simulink model "PedalBoard"  (R2018b)
settings: Solver=VariableStepAuto  StartTime=0.0  StopTime=10.0  RelTol=1e-3
libraries: canoelib x4
settings Model: Creator=jackb  LastModifiedBy=jackb

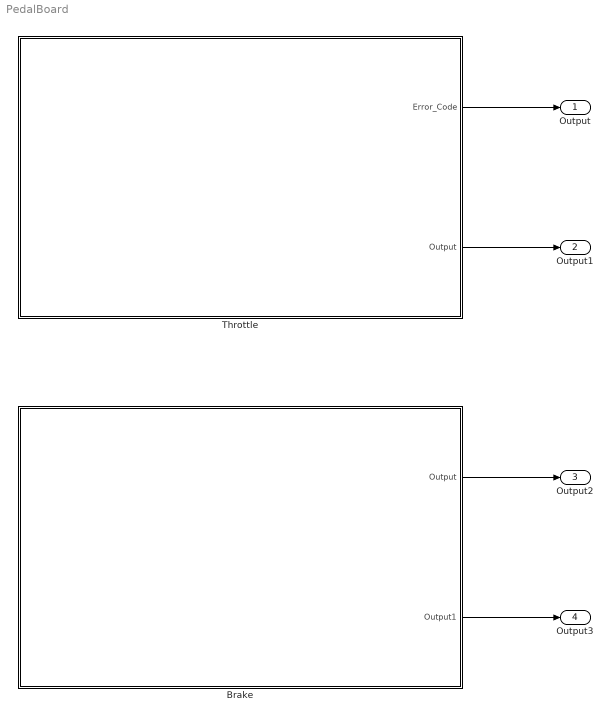
== system PedalBoard ==
  Brake : Subsystem
  "Throttle " : Subsystem
  Output : Outport
  Output1 : Outport  Port=2
  Output2 : Outport  Port=3
  Output3 : Outport  Port=4
  wires:
  "Throttle "/2(Output) -> Output1/1
  "Throttle "/1(Error_Code) -> Output/1
  Brake/1(Output) -> Output2/1
  Brake/2(Output1) -> Output3/1

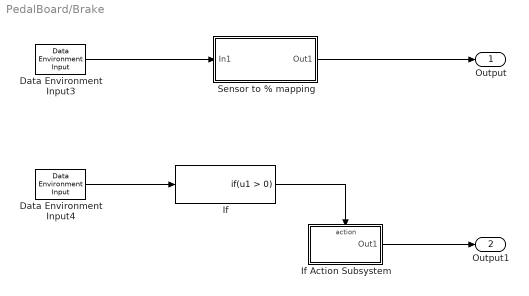
== system PedalBoard/Brake ==
  Data Environment Input3 : canoelib/CANoe I//O/Data Environment Input  envName=Brk_Pos  editSampleTime=0  dataType=Default  dataTypeDB=double
      settings: AttributesFormatString=%<envName>  SourceProductName=Vector CANoe
  Data Environment Input4 : canoelib/CANoe I//O/Data Environment Input  envName=Brk_Ovr_Trv  editSampleTime=0  dataType=Default  dataTypeDB=int32
      settings: AttributesFormatString=%<envName>  SourceProductName=Vector CANoe
  If : If  ShowElse=off
  If Action Subsystem : Subsystem  TreatAsAtomicUnit=on
  Sensor to % mapping : Subsystem
  Output : Outport
  Output1 : Outport  Port=2
  wires:
  Data Environment Input3/1 -> Sensor to % mapping/1(In1)
  Sensor to % mapping/1(Out1) -> Output/1
  Data Environment Input4/1 -> If/1
  If/1 -> If Action Subsystem/Action
  If Action Subsystem/1(Out1) -> Output1/1

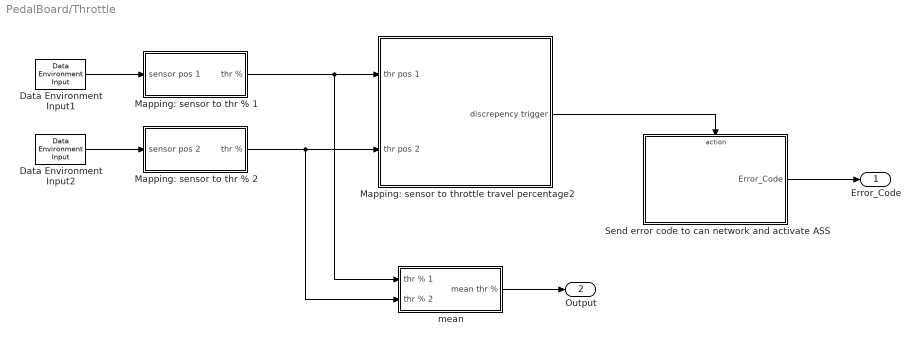
== system PedalBoard/Throttle  ==
  Data Environment Input1 : canoelib/CANoe I//O/Data Environment Input  envName=Thr_Pos_1  editSampleTime=0  dataType=Default  dataTypeDB=double
      settings: AttributesFormatString=%<envName>  SourceProductName=Vector CANoe
  Data Environment Input2 : canoelib/CANoe I//O/Data Environment Input  envName=Thr_Pos_2  editSampleTime=0  dataType=Default  dataTypeDB=double
      settings: AttributesFormatString=%<envName>  SourceProductName=Vector CANoe
  Mapping: sensor to thr % 1 : Subsystem
  Mapping: sensor to thr % 2 : Subsystem
  Mapping: sensor to throttle travel percentage2 : Subsystem
  Send error code to can network and activate ASS : Subsystem  TreatAsAtomicUnit=on
  mean : Subsystem
  Error_Code : Outport
  Output : Outport  Port=2
  wires:
  Data Environment Input2/1 -> Mapping: sensor to thr % 2/1("sensor pos 2 ")
  Mapping: sensor to thr % 2/1("thr % ") -> mean/2("thr % 2 "), Mapping: sensor to throttle travel percentage2/2(thr pos 2)
  Mapping: sensor to thr % 1/1("thr % ") -> mean/1(thr % 1), Mapping: sensor to throttle travel percentage2/1("thr pos 1 ")
  Mapping: sensor to throttle travel percentage2/1(discrepency trigger) -> Send error code to can network and activate ASS/Action
  Data Environment Input1/1 -> Mapping: sensor to thr % 1/1("sensor pos 1 ")
  mean/1("mean thr % ") -> Output/1
  Send error code to can network and activate ASS/1("Error_Code ") -> Error_Code/1

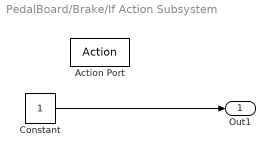
== system PedalBoard/Brake/If Action Subsystem ==
  Action Port : ActionPort
  Constant : Constant
  Out1 : Outport
  wires:
  Constant/1 -> Out1/1

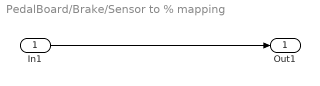
== system PedalBoard/Brake/Sensor to % mapping ==
  In1 : Inport
  Out1 : Outport
  wires:
  In1/1 -> Out1/1

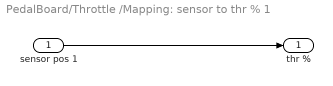
== system PedalBoard/Throttle /Mapping: sensor to thr % 1 ==
  "sensor pos 1 " : Inport
  "thr % " : Outport
  wires:
  "sensor pos 1 "/1 -> "thr % "/1

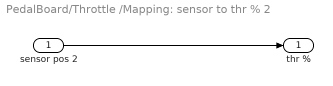
== system PedalBoard/Throttle /Mapping: sensor to thr % 2 ==
  "sensor pos 2 " : Inport
  "thr % " : Outport
  wires:
  "sensor pos 2 "/1 -> "thr % "/1

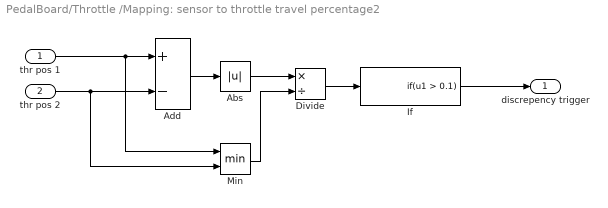
== system PedalBoard/Throttle /Mapping: sensor to throttle travel percentage2 ==
  "thr pos 1 " : Inport
  thr pos 2 : Inport  Port=2
  Abs : Abs
  Add : Sum  Inputs=+-
  Divide : Product  Inputs=*/
  If : If  IfExpression=u1 > 0.1  ShowElse=off
  Min : MinMax  Inputs=2
  discrepency trigger : Outport
  wires:
  "thr pos 1 "/1 -> Min/1, Add/1
  thr pos 2/1 -> Min/2, Add/2
  Add/1 -> Abs/1
  Abs/1 -> Divide/1
  Min/1 -> Divide/2
  Divide/1 -> If/1
  If/1 -> discrepency trigger/1

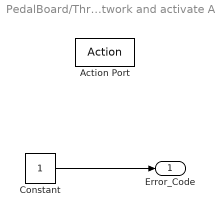
== system PedalBoard/Throttle /Send error code to can network and activate ASS ==
  Action Port : ActionPort
  Constant : Constant
  "Error_Code " : Outport
  wires:
  Constant/1 -> "Error_Code "/1

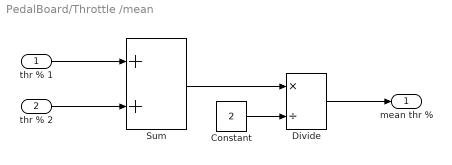
== system PedalBoard/Throttle /mean ==
  thr % 1 : Inport
  "thr % 2 " : Inport  Port=2
  Constant : Constant  Value=2
  Divide : Product  Inputs=*/
  Sum : Sum
  "mean thr % " : Outport
  wires:
  "thr % 2 "/1 -> Sum/2
  thr % 1/1 -> Sum/1
  Sum/1 -> Divide/1
  Constant/1 -> Divide/2
  Divide/1 -> "mean thr % "/1
